simulink model "SingleKernel"  (R2019b)
settings: Solver=VariableStepAuto  StartTime=0.0  StopTime=4098*4  RelTol=1e-3
PreLoadFcn:
  | load taps
undefined symbols (not defined in the file or in its folder): FIR_SingleStream, SingleStream, xc7vx485tffg1157
libraries: ModelComposer x4, dspsrcs4 x2
settings Model: Creator=abehbood  LastModifiedBy=abehbood

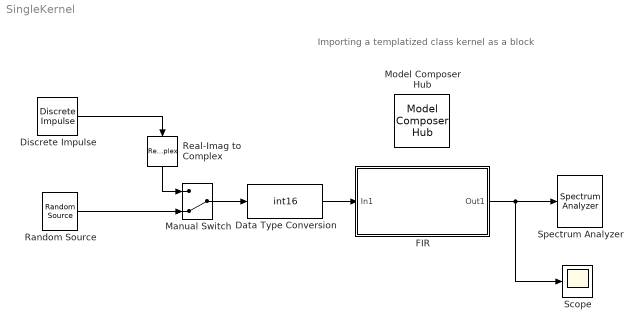
== system SingleKernel ==
  note: Importing a templatized class kernel as a block
  Data Type Conversion : DataTypeConversion  OutDataTypeStr=int16
  Discrete Impulse : dspsrcs4/Discrete  Impulse  Delay=0  SampleTime=1  FrameSample=512  OutputFrames=off  dataType=double  isSigned=on  wordLen=16  udDataType=sfix(16)  fracBitsMode=Best precision  numFracBits=15  OutDataTypeStr=double  LastOutDataTypeStr=double
  FIR : Subsystem
  Manual Switch : ManualSwitch  CurrentSetting=0
  Model Composer Hub : ModelComposer/Model Composer Hub  CodeGeneration=off  SubsystemName=FIR  TargetDirectory=./code  ExportType=AI Engines  IpVendor=xilinx.com  IpLibrary=hls  IpVersion=1.0  IpHWLanguage=Verilog  AieCompilerOptions={}  CreateTestbench=on  TestbenchStackSize=10  RunAieSim=on  AieSimTimeout=50000  LaunchVitisAnalyzer=off  RunX86Sim=off  X86SimTimeout=10  ProjDevice=xc7vx485tffg1157-1  ProjDevicePart=xc7vx485tffg1157-1  SamplePeriod=-1  ClockFrequency=200  DataPathParallelism=1
  Random Source : dspsrcs4/Random Source  SrcType=Uniform  NormMethod=Ziggurat  CltLength=12  MinVal=-1  MaxVal=1  MeanVal=0  VarVal=1  RepMode=Not repeatable  rawSeed=1  IsInherit=off  SampMode=Discrete  SampTime=1  SampFrame=512  DataType=Double  OutComplex=Complex  OutputFrames=off
  Real-Imag to Complex : RealImagToComplex  Input=Real
  Scope : Scope
  Spectrum Analyzer : SpectrumAnalyzer
  wires:
  Data Type Conversion/1 -> FIR/1(In1)
  FIR/1(Out1) -> Scope/1, Spectrum Analyzer/1
  Manual Switch/1 -> Data Type Conversion/1
  Random Source/1 -> Manual Switch/2
  Discrete Impulse/1 -> Real-Imag to Complex/1
  Real-Imag to Complex/1 -> Manual Switch/1

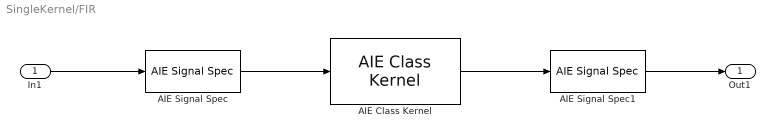
== system SingleKernel/FIR ==
  In1 : Inport
  AIE Class Kernel : ModelComposer/AIE Class Kernel  KernelAllAttrs=|  PortNames={'sin'; 'sout'}  PortSerializedTypes={'{P{Tinput_stream{1{t{Scint16}}}}}'; '{P{Toutput_stream{1{t{Scint16}}}}}'}  PortWindowSizes={0.000000000000000000e+00; 0.000000000000000000e+00}  PortWindowMargins={0.000000000000000000e+00; 0.000000000000000000e+00}  PortSynchronicities={'auto'; 'auto'}  PortSignalSizes={0.000000000000000000e+00; 5.120000000000000000e+02}  ClassTemplateSpecKind=implicit  ClassTemplateParamNames={'NSamples'; 'ShiftAcc'}  ClassTemplateParamKinds={'nontype'; 'nontype'}  ClassTemplateParamTypes={'int'; 'int'}  ClassTemplateParamValues={'512', '0'}  ClassCtorParamNames={'taps'}  ClassCtorParamSerializedTypes={'{R{Q1{C{Scint16}32}}}'}  ClassCtorParamValues={'[-82-253i;0-204i;11-35i;-198+273i;-642+467i;-1026+333i;-927;-226-73i;643+467i;984+1355i;550+1691i;0+647i;538-1656i;2860-3936i;6313-4587i;9113-2961i;9582;7421+2411i;3936+2860i;1023+1409i;-200-615i;0-1778i;517-1592i;467-643i;-192+140i;-882+287i;-1079;-755-245i;-273-198i;22+30i;63+194i;0+266i]'}  ClassIndex=1  ClassCtorIndex=1  ClassTabVisible=on  ClassTemplateParamsVisible=on  ClassCtorDeclVisible=on  ClassCtorParamsVisible=on  FunctionTabVisible=on  FunctionDecl=|  PortAttrs={ 'input', 'sin', 'input_stream_cint16 *', '', '', '', ''; 'output', 'sout', 'output_stream_cint16 *', '', '', '', '512' }  PortAttrsEnables={'off', 'off', 'off', 'off', 'off', 'off', 'off';'off', 'off', 'off', 'off', 'off', 'off', 'on'}  ClassDeclTypeOptions=|  ClassDecl=|  ClassTemplateParams={ 'NSamples', 'int', '512'; 'ShiftAcc', 'int', '0' }  ClassTemplateParamsEnables={'off', 'off', 'on';'off', 'off', 'on'}  ClassCtorDeclTypeOptions=C[1 1]@t48@FIR_SingleStream(cint16 const ( & taps ) [ 32 ])  ClassCtorDecl=FIR_SingleStream(cint16 const ( & taps ) [ 32 ])  ClassCtorParams={ 'taps', 'cint16 const ( &) [ 32 ]', 'taps' }  KernelHeaderFile=src/aie_kernels/FirSingleStream.h  KernelClassName=SingleStream::FIR_SingleStream  KernelFunction=filter  KernelSourceFile=src/aie_kernels/FirSingleStream.cpp  KernelSearchPaths={}  PreProcOptions={}  CoreRuntimeRatio=0.9  KernelLocSpec=off  ColRowLocation=[0 0]
      KernelAllAttrs=|
      | s[12;12;9;9;19;14;21;23;24;21;12;24;26;26;26;27;28;9;21;23;23;23;24;25;14;19;19;29]@FunctionNameDeclFileNamePortNamesPortTypesPortSerializedTypesPortDirectionsPortWindowSizeEnablesPortWindowMarginEnablesPortSynchronicityEnablesPortSignalSizeEnablesFunctionDeclFunctionTemplateSpecKindFunctionTemplateParamNamesFunctionTemplateParamKindsFunctionTemplateParamTypesFunctionTemplateParamValuesFunctionTemplateParamEnablesClassDeclClassTemplateSpecKindClassTemplateParamNamesClassTemplateParamKindsClassTemplateParamTypesClassTemplateParamValuesClassTemplateParamEnablesClassCtorDeclsClassCtorParamNamesClassCtorParamTypesClassCtorParamSerializedTypes[1 1]@C[28 1]@t6@filtert39@../../src/aie_kernels/FirSingleStream.hC[2 1]@t3@sint4@soutC[2 1]@t21@input_stream_cint16 *t22@output_stream_cint16 *C[2 1]@t33@{P{Tinput_stream{1{t{Scint16}}}}}t34@{P{Toutput_stream{1{t{Scint16}}}}}C[2 1]@t5@inputt6@outputC[2 1]@l0@l0@C[2 1]@l0@l0@C[2 1]@l0@l0@C[2 1]@l0@l1@t155@namespace SingleStream {
      | template < int NSamples, int ShiftAcc > 
      | void FIR_SingleStream::
      | filter(input_stream_cint16 * sin, output_stream_cint16 * sout);
      | }t4@nonee[0 1]@e[0 1]@e[0 1]@e[0 1]@e[0 1]@t90@namespace SingleStream {
      | template < int NSamples, int ShiftAcc > class FIR_SingleStream;
      | }t8@implicitC[2 1]@t8@NSamplest8@ShiftAccC[2 1]@t7@nontypet7@nontypeC[2 1]@t3@intt3@intC[2 1]@nnC[2 1]@l1@l1@C[1 1]@t48@FIR_SingleStream(cint16 const ( & taps ) [ 32 ])C[1 1]@C[1 1]@t4@tapsC[1 1]@C[1 1]@t24@cint16 const ( &) [ 32 ]C[1 1]@C[1 1]@t21@{R{Q1{C{Scint16}32}}}
      FunctionDecl=|
      | namespace SingleStream {
      | template < int NSamples, int ShiftAcc > 
      | void FIR_SingleStream::
      | filter(input_stream_cint16 * sin, output_stream_cint16 * sout);
      | }
      ClassDeclTypeOptions=|
      | C[1 1]@t90@namespace SingleStream {
      | template < int NSamples, int ShiftAcc > class FIR_SingleStream;
      | }
      ClassDecl=|
      | namespace SingleStream {
      | template < int NSamples, int ShiftAcc > class FIR_SingleStream;
      | }
  AIE Signal Spec : ModelComposer/AIE Signal Spec  DestFifoDepth=0  SrcFifoDepth=0  PlioWidth=64  PlioFreqSpec=on  PlioFreq=500
  AIE Signal Spec1 : ModelComposer/AIE Signal Spec  DestFifoDepth=0  SrcFifoDepth=0  PlioWidth=64  PlioFreqSpec=on  PlioFreq=500
  Out1 : Outport
  wires:
  AIE Class Kernel/1 -> AIE Signal Spec1/1
  In1/1 -> AIE Signal Spec/1
  AIE Signal Spec/1 -> AIE Class Kernel/1
  AIE Signal Spec1/1 -> Out1/1
